simulink model "simulate"  (R2023a)
settings: Solver=VariableStepAuto  StartTime=0.0  StopTime=20.0  RelTol=1e-3
settings Model: Creator=zhs20  LastModifiedBy=zhs20

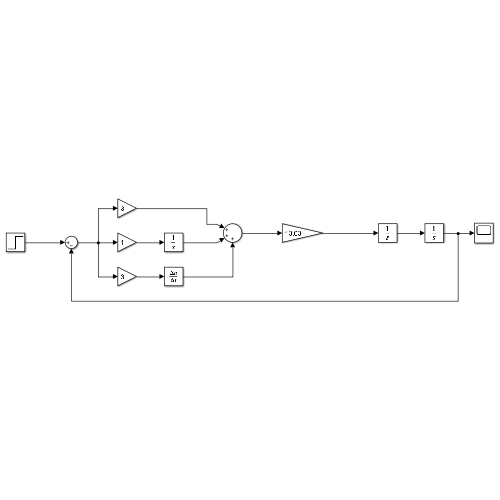
[thumbnail: Simulink's stored preview of the top-level diagram]
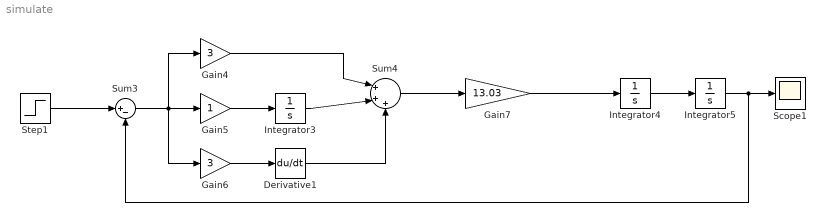
== system simulate ==
  Derivative1 : Derivative
  Gain4 : Gain  Gain=3
  Gain5 : Gain
  Gain6 : Gain  Gain=3
  Gain7 : Gain  Gain=13.03
  Integrator3 : Integrator
  Integrator4 : Integrator
  Integrator5 : Integrator
  Scope1 : Scope
  Step1 : Step  After=0.3  SampleTime=0
  Sum3 : Sum  Inputs=|+-
  Sum4 : Sum  Inputs=|+++
  wires:
  Gain7/1 -> Integrator4/1
  Gain6/1 -> Derivative1/1
  Gain4/1 -> Sum4/1
  Derivative1/1 -> Sum4/3
  Gain5/1 -> Integrator3/1
  Integrator3/1 -> Sum4/2
  Step1/1 -> Sum3/1
  Integrator4/1 -> Integrator5/1
  Sum3/1 -> Gain4/1, Gain5/1, Gain6/1
  Sum4/1 -> Gain7/1
  Integrator5/1 -> Scope1/1, Sum3/2
